simulink library "periodicCtrlExpAllocate"  (R2020a)
settings: Solver=VariableStepAuto  StartTime=0.0  StopTime=10.0  RelTol=1e-3
undefined symbols (not defined in the file or in its folder): fltCtrl, initializeBussesFromBlock
libraries: dspsigops x2, filteredPIDController_ul x2, eulAng2RotMat_ul x1
settings Model: Creator=jcreed2  LastModifiedBy=andre

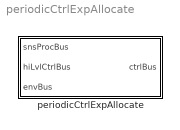
== system periodicCtrlExpAllocate ==
  periodicCtrlExpAllocate : Subsystem  LoadFcn=initializeBussesFromBlock(gcb)  InitFcn=initializeBussesFromBlock(gcb)  mask{fltCtrl=fltCtrl}
      mask prompts: fltCtrl "Controller Model"

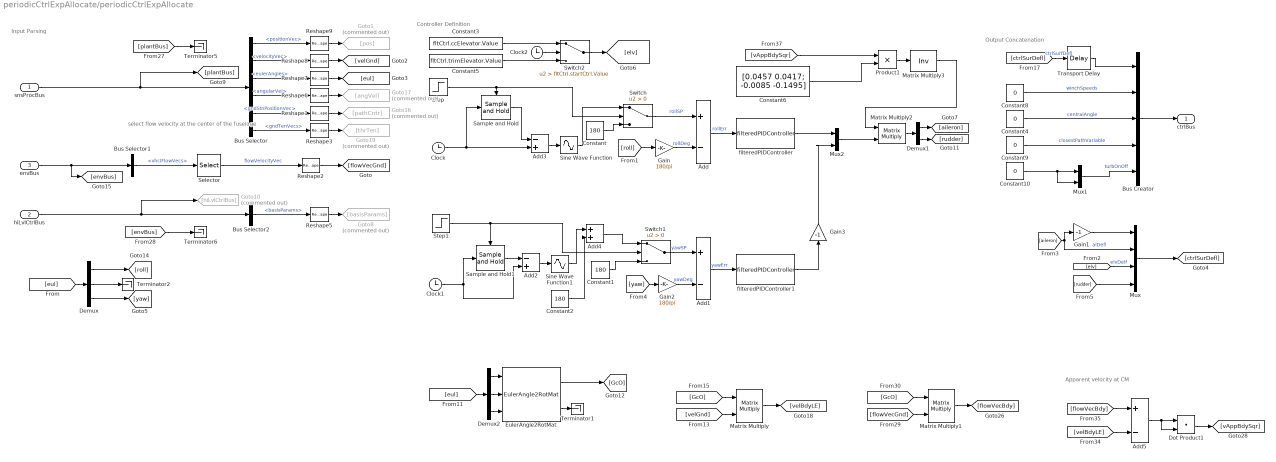
== system periodicCtrlExpAllocate/periodicCtrlExpAllocate ==
  note: Controller Definition
  note: select flow velocity at the center of the fuselage
  note: Input Parsing
  note: Output Concatenation
  note: Apparent velocity at CM
  snsProcBus : Inport  OutDataTypeStr=Bus: sensorsProcessingBus
  hiLvlCtrlBus : Inport  Port=2  OutDataTypeStr=Bus: hiLvlCtrlBus
  envBus : Inport  Port=3  OutDataTypeStr=Bus: envBus
  Add : Sum  Inputs=+-
  Add1 : Sum  Inputs=+-
  Add2 : Sum  Inputs=-+
  Add3 : Sum  Inputs=-+
  Add4 : Sum
  Add5 : Sum  Inputs=+-
  Bus Creator : BusCreator  Inputs=5  OutDataTypeStr=Bus: fltCtrlBus
      settings: InheritFromInputs=off
  Bus Selector : BusSelector  OutputSignals=positionVec,velocityVec,eulerAngles,angularVel,gndStnPositionVec,gndTenVecs
  Bus Selector1 : BusSelector  OutputSignals=vhclFlowVecs
  Bus Selector2 : BusSelector  OutputSignals=basisParams
  Clock : Clock
  Clock1 : Clock
  Clock2 : Clock
  Constant : Constant  Value=180
  Constant1 : Constant  Value=180
  Constant{4,8..10} (4 alike) : Constant  Value=0
  Constant2 : Constant  Value=180
  Constant3 : Constant  Value=fltCtrl.ccElevator.Value
  Constant5 : Constant  Value=fltCtrl.trimElevator.Value
  Constant6 : Constant  Value=[0.0457 0.0417; -0.0085 -0.1495]
  Demux : Demux  Outputs=3
  Demux1 : Demux  Outputs=2
  Demux2 : Demux  Outputs=3
  Dot Product1 : DotProduct  InputSameDT=on  OutDataTypeStr=Inherit: Inherit via internal rule
  EulerAngle2RotMat : eulAng2RotMat_ul/EulerAngle2RotMat  SystemSampleTime=-1  Latency=0  AutoFrameSizeCalculation=off
  Gain : Gain  Gain=180/pi
  Gain1 : Gain  Gain=-1
  Gain2 : Gain  Gain=180/pi
  Gain3 : Gain  Gain=-1
  Goto1 : Goto  Commented=on  GotoTag=pos
  Goto10 : Goto  Commented=on  GotoTag=hiLvlCtrlBus
  Goto16 : Goto  Commented=on  GotoTag=pathCntr
  Goto17 : Goto  Commented=on  GotoTag=angVel
  Goto19 : Goto  Commented=on  GotoTag=thrTen
  Goto8 : Goto  Commented=on  GotoTag=basisParams
  Matrix Multiply : Product  Multiplication=Matrix(*)
  Matrix Multiply1 : Product  Multiplication=Matrix(*)
  Matrix Multiply2 : Product  Multiplication=Matrix(*)
  Matrix Multiply3 : Product  Inputs=/  Multiplication=Matrix(*)
  Mux : Mux
  Mux1 : Mux  Inputs=2
  Mux2 : Mux  Inputs=2
  Product1 : Product
  Reshape{1..3,5..9} (8 alike) : Reshape  OutputDimensionality=Column vector (2-D)
  Sample and Hold : dspsigops/Sample and Hold  trig=Rising edge  initCond=0  latchinput=off
  Sample and Hold1 : dspsigops/Sample and Hold  trig=Rising edge  initCond=0  latchinput=off
  Selector : Selector  NumberOfDimensions=2  InputPortWidth=3  IndexOptions=Select all,Index vector (dialog)  Indices=[1 3],5  OutputSizes=1,1
  Sine Wave Function : Sin  TimeSource=Use external signal  Amplitude=fltCtrl.rollAmp.Value  Bias=180  Frequency=fltCtrl.frequency.Value  Phase=fltCtrl.rollPhase.Value  SampleTime=0
  Sine Wave Function1 : Sin  TimeSource=Use external signal  Amplitude=fltCtrl.yawAmp.Value  Frequency=fltCtrl.frequency.Value  Phase=fltCtrl.yawPhase.Value  SampleTime=0
  Step : Step  Time=fltCtrl.startCtrl.Value  SampleTime=0
  Step1 : Step  Time=fltCtrl.startCtrl.Value  SampleTime=0
  Switch : Switch  Criteria=u2 > Threshold
  Switch1 : Switch  Criteria=u2 > Threshold
  Switch2 : Switch  Criteria=u2 > Threshold  Threshold=fltCtrl.startCtrl.Value
  Terminator{1..2,5..6} (4 alike) : Terminator
  Transport Delay : TransportDelay  DelayTime=.060
  filteredPIDController : filteredPIDController_ul/filteredPIDController  kp=fltCtrl.rollCtrl.kp.Value  ki=fltCtrl.rollCtrl.ki.Value  kd=fltCtrl.rollCtrl.kd.Value  Value=fltCtrl.rollCtrl.tau.Value  externalReset=none
  filteredPIDController1 : filteredPIDController_ul/filteredPIDController  kp=fltCtrl.yawCtrl.kp.Value  ki=fltCtrl.yawCtrl.ki.Value  kd=fltCtrl.yawCtrl.kd.Value  Value=fltCtrl.yawCtrl.tau.Value  externalReset=none
  ctrlBus : Outport  OutDataTypeStr=Bus: fltCtrlBus  VectorParamsAs1DForOutWhenUnconnected=off
  wires:
  Reshape1/1 -> Goto16/1
  Reshape9/1 -> Goto1/1
  Bus Selector/5 -> Reshape1/1  "<gndStnPositionVec>"
  Bus Selector/3 -> Reshape7/1  "<eulerAngles>"
  Demux/2 -> Terminator2/1
  Gain1/1 -> Mux/1
  [envBus] -> Terminator6/1
  Reshape3/1 -> Goto19/1
  [rudder] -> Mux/4
  Constant5/1 -> Switch2/3
  Reshape5/1 -> Goto8/1
  envBus/1 -> [envBus], Bus Selector1/1
  Bus Creator/1 -> ctrlBus/1
  Bus Selector/1 -> Reshape9/1  "<positionVec>"
  Constant8/1 -> Bus Creator/2  "winchSpeeds"
  Bus Selector/4 -> Reshape6/1  "<angularVel>"
  Reshape6/1 -> Goto17/1
  Bus Selector2/1 -> Reshape5/1  "<basisParams>"
  Bus Selector/2 -> Reshape8/1  "<velocityVec>"
  [aileron] -> Mux/2, Gain1/1  "alDefl"
  Reshape2/1 -> [flowVecGnd]
  [ctrlSurDefl] -> Transport Delay/1  "ctrlSurfDefl"
  [elv] -> Mux/3  "elvDelf"
  [plantBus] -> Terminator5/1
  Reshape7/1 -> [eul]
  Selector/1 -> Reshape2/1  "flowVelocityVec"
  [eul] -> Demux/1
  Bus Selector/6 -> Reshape3/1  "<gndTenVecs>"
  Demux/1 -> [roll]
  Demux/3 -> [yaw]
  Reshape8/1 -> [velGnd]
  Bus Selector1/1 -> Selector/1  "<vhclFlowVecs>"
  [roll] -> Gain/1
  Add/1 -> filteredPIDController/1  "rollErr"
  Gain/1 -> Add/2  "rollDeg"
  Clock/1 -> Add3/2, Sample and Hold/1
  Mux/1 -> [ctrlSurDefl]
  Clock2/1 -> Switch2/2
  Switch2/1 -> [elv]
  Constant3/1 -> Switch2/1
  Sample and Hold/1 -> Add3/1
  Add3/1 -> Sine Wave Function/1
  Sine Wave Function/1 -> Switch/1
  Step/1 -> Switch/2, Sample and Hold/Trigger
  Constant/1 -> Switch/3
  Switch/1 -> Add/1  "rollSP"
  Constant4/1 -> Bus Creator/3  "centralAngle"
  Constant9/1 -> Bus Creator/4  "closestPathVariable"
  Constant10/1 -> Mux1/2, Mux1/1
  Mux1/1 -> Bus Creator/5  "turbOnOff"
  Step1/1 -> Switch1/2, Sample and Hold1/Trigger
  Constant1/1 -> Switch1/3
  Switch1/1 -> Add1/1  "yawSP"
  Add2/1 -> Sine Wave Function1/1
  Gain2/1 -> Add1/2  "yawDeg"
  [yaw] -> Gain2/1
  Sample and Hold1/1 -> Add2/1
  Clock1/1 -> Sample and Hold1/1, Add2/2
  Add1/1 -> filteredPIDController1/1  "yawErr"
  snsProcBus/1 -> Bus Selector/1, [plantBus]
  hiLvlCtrlBus/1 -> Goto10/1, Bus Selector2/1
  filteredPIDController/1 -> Mux2/1
  filteredPIDController1/1 -> Gain3/1
  Transport Delay/1 -> Bus Creator/1
  Sine Wave Function1/1 -> Add4/1
  Constant2/1 -> Add4/2
  Add4/1 -> Switch1/1
  [vAppBdySqr] -> Product1/1
  Product1/1 -> Matrix Multiply3/1
  Constant6/1 -> Product1/2
  Matrix Multiply3/1 -> Matrix Multiply2/1
  Mux2/1 -> Matrix Multiply2/2
  Matrix Multiply2/1 -> Demux1/1
  Demux1/1 -> [aileron]
  Demux1/2 -> [rudder]
  Add5/1 -> Dot Product1/2, Dot Product1/1
  [flowVecBdy] -> Add5/1
  EulerAngle2RotMat/1 -> [GcO]
  Demux2/2 -> EulerAngle2RotMat/2
  Demux2/1 -> EulerAngle2RotMat/1
  Demux2/3 -> EulerAngle2RotMat/3
  [velGnd] -> Matrix Multiply/2
  [eul] -> Demux2/1
  Matrix Multiply1/1 -> [flowVecBdy]
  Matrix Multiply/1 -> [velBdyLE]
  [flowVecGnd] -> Matrix Multiply1/2
  [GcO] -> Matrix Multiply1/1
  [GcO] -> Matrix Multiply/1
  [velBdyLE] -> Add5/2
  EulerAngle2RotMat/2 -> Terminator1/1
  Dot Product1/1 -> [vAppBdySqr]
  Gain3/1 -> Mux2/2
